simulink subsystem "DriverHEVPowerSplit_refsub"  (R2020b)
settings: Solver=VariableStepAuto  StartTime=0.0  StopTime=10.0  RelTol=1e-3
undefined symbols (not defined in the file or in its folder): driver, initial
libraries: EVComponents_utility_lib x3, simulink x2
settings Model: Creator=isaacito  LastModifiedBy=isaacito

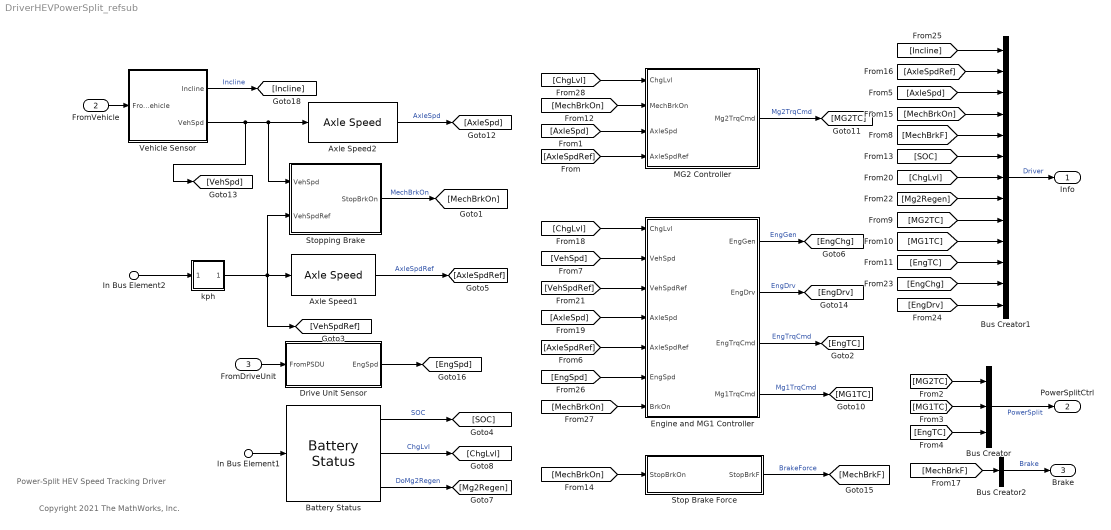
== system DriverHEVPowerSplit_refsub ==
  note: Power-Split HEV Speed Tracking Driver
  note: Copyright 2021 The MathWorks, Inc.
  In Bus Element1 : Inport  PortName=FromBattery  Element=Current
  FromVehicle : Inport  Port=2
  FromDriveUnit : Inport  Port=3
  In Bus Element2 : Inport  Port=4  PortName=FromDrvPattern  Element=VehSpdRef
      settings: AttributesFormatString=%<Unit>
  Axle Speed1 : EVComponents_utility_lib/Axle Speed  Value=driver.tireRadius_m
  Axle Speed2 : EVComponents_utility_lib/Axle Speed  Value=driver.tireRadius_m
  Battery Status : EVComponents_utility_lib/Battery Status  capacity_Ahr=driver.hvbattCapacity_Ahr  initial_SOC_pct=initial.driverHVBattSOC_pct  SocHigh=driver.hvbattSocHighMid_pct  SocLow=driver.hvbattSocMidLow_pct  SocEmpty=driver.hvbattSocLowEmpty_pct
  Bus Creator : BusCreator  Inputs=3
  Bus Creator1 : BusCreator  Inputs=13
  Bus Creator2 : BusCreator  Inputs=1
  Drive Unit Sensor : Subsystem
  Engine and MG1 Controller : Subsystem
  MG2 Controller : Subsystem
  Stop Brake Force : Subsystem
  Stopping Brake : Subsystem
  Vehicle Sensor : Subsystem
  kph : Subsystem
  Info : Outport
  PowerSplitCtrl : Outport  Port=2
  Brake : Outport  Port=3
  wires:
  In Bus Element2/1 -> kph/1(In1)
  FromVehicle/1 -> Vehicle Sensor/1(FromVehicle)
  Vehicle Sensor/2(VehSpd) -> Axle Speed2/1, Stopping Brake/1(VehSpd), [VehSpd]
  Battery Status/1 -> [SOC]  "SOC"
  [SOC] -> Bus Creator1/6
  [Mg2Regen] -> Bus Creator1/8
  [ChgLvl] -> Bus Creator1/7
  [MechBrkOn] -> Bus Creator1/4
  [AxleSpd] -> Bus Creator1/3
  Engine and MG1 Controller/4(Mg1TrqCmd) -> [MG1TC]  "Mg1TrqCmd"
  [VehSpdRef] -> Engine and MG1 Controller/3(VehSpdRef)
  [AxleSpdRef] -> Engine and MG1 Controller/5(AxleSpdRef)
  [AxleSpd] -> Engine and MG1 Controller/4(AxleSpd)
  [AxleSpdRef] -> Bus Creator1/2
  Bus Creator1/1 -> Info/1  "Driver"
  [MG1TC] -> Bus Creator1/10
  [MG2TC] -> Bus Creator1/9
  [MechBrkF] -> Bus Creator1/5
  [EngTC] -> Bus Creator1/11
  [VehSpd] -> Engine and MG1 Controller/2(VehSpd)
  Axle Speed2/1 -> [AxleSpd]  "AxleSpd"
  Battery Status/3 -> [Mg2Regen]  "DoMg2Regen"
  Battery Status/2 -> [ChgLvl]  "ChgLvl"
  Engine and MG1 Controller/3(EngTrqCmd) -> [EngTC]  "EngTrqCmd"
  [ChgLvl] -> Engine and MG1 Controller/1(ChgLvl)
  [EngTC] -> Bus Creator/3
  [MG1TC] -> Bus Creator/2
  [MG2TC] -> Bus Creator/1
  Bus Creator/1 -> PowerSplitCtrl/1  "PowerSplit"
  Axle Speed1/1 -> [AxleSpdRef]  "AxleSpdRef"
  [MechBrkF] -> Bus Creator2/1
  Bus Creator2/1 -> Brake/1  "Brake"
  In Bus Element1/1 -> Battery Status/1
  Engine and MG1 Controller/1(EngGen) -> [EngChg]  "EngGen"
  Engine and MG1 Controller/2(EngDrv) -> [EngDrv]  "EngDrv"
  [EngChg] -> Bus Creator1/12
  [EngDrv] -> Bus Creator1/13
  [EngSpd] -> Engine and MG1 Controller/6(EngSpd)
  [MechBrkOn] -> Engine and MG1 Controller/7(BrkOn)
  FromDriveUnit/1 -> Drive Unit Sensor/1(FromPSDU)
  Drive Unit Sensor/1(EngSpd) -> [EngSpd]
  [MechBrkOn] -> MG2 Controller/2(MechBrkOn)
  [AxleSpd] -> MG2 Controller/3(AxleSpd)
  [AxleSpdRef] -> MG2 Controller/4(AxleSpdRef)
  [MechBrkOn] -> Stop Brake Force/1(StopBrkOn)
  Vehicle Sensor/1(Incline) -> [Incline]  "Incline"
  MG2 Controller/1(Mg2TrqCmd) -> [MG2TC]  "Mg2TrqCmd"
  Stopping Brake/1(StopBrkOn) -> [MechBrkOn]  "MechBrkOn"
  Stop Brake Force/1(StopBrkF) -> [MechBrkF]  "BrakeForce"
  [Incline] -> Bus Creator1/1
  [ChgLvl] -> MG2 Controller/1(ChgLvl)
  kph/1(Out1) -> Axle Speed1/1, [VehSpdRef], Stopping Brake/2(VehSpdRef)

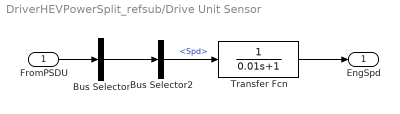
== system DriverHEVPowerSplit_refsub/Drive Unit Sensor ==
  FromPSDU : Inport
  Bus Selector : BusSelector  OutputSignals=eng  OutputAsBus=on
  Bus Selector2 : BusSelector  OutputSignals=Spd
  Transfer Fcn : TransferFcn  Denominator=[0.01 1]
  EngSpd : Outport  Unit=rpm
      settings: AttributesFormatString=%<Unit>
  wires:
  Bus Selector/1 -> Bus Selector2/1
  Transfer Fcn/1 -> EngSpd/1
  FromPSDU/1 -> Bus Selector/1
  Bus Selector2/1 -> Transfer Fcn/1  "<Spd>"

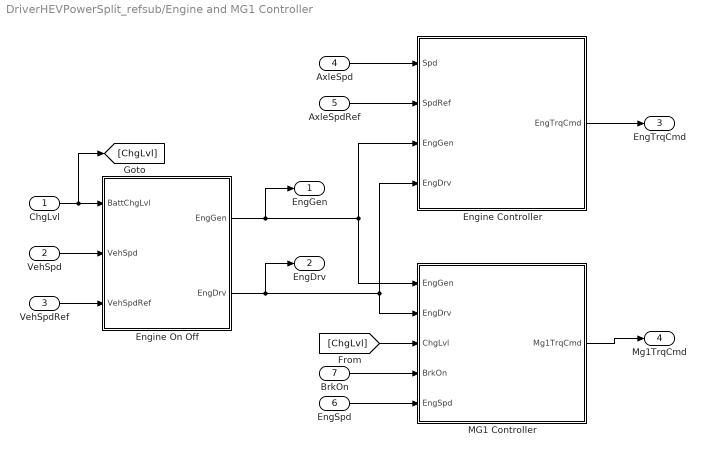
== system DriverHEVPowerSplit_refsub/Engine and MG1 Controller ==
  ChgLvl : Inport
  VehSpd : Inport  Port=2  Unit=km/hr
      settings: AttributesFormatString=%<Unit>
  VehSpdRef : Inport  Port=3  Unit=km/hr
      settings: AttributesFormatString=%<Unit>
  AxleSpd : Inport  Port=4  Unit=rpm
      settings: AttributesFormatString=%<Unit>
  AxleSpdRef : Inport  Port=5  Unit=rpm
      settings: AttributesFormatString=%<Unit>
  EngSpd : Inport  Port=6  Unit=rpm
      settings: AttributesFormatString=%<Unit>
  BrkOn : Inport  Port=7
  Engine Controller : Subsystem
  Engine On Off : Stateflow chart  TreatAsAtomicUnit=on
  MG1 Controller : Subsystem
  EngGen : Outport
  EngDrv : Outport  Port=2
  EngTrqCmd : Outport  Port=3  Unit=N*m
      settings: AttributesFormatString=%<Unit>
  Mg1TrqCmd : Outport  Port=4  Unit=N*m
      settings: AttributesFormatString=%<Unit>
  wires:
  VehSpd/1 -> Engine On Off/2(VehSpd)
  ChgLvl/1 -> [ChgLvl], Engine On Off/1(BattChgLvl)
  VehSpdRef/1 -> Engine On Off/3(VehSpdRef)
  Engine On Off/1(EngGen) -> MG1 Controller/1(EngGen), Engine Controller/3(EngGen), EngGen/1
  Engine On Off/2(EngDrv) -> EngDrv/1, Engine Controller/4(EngDrv), MG1 Controller/2(EngDrv)
  AxleSpd/1 -> Engine Controller/1(Spd)
  AxleSpdRef/1 -> Engine Controller/2(SpdRef)
  Engine Controller/1(EngTrqCmd) -> EngTrqCmd/1
  BrkOn/1 -> MG1 Controller/4(BrkOn)
  EngSpd/1 -> MG1 Controller/5(EngSpd)
  MG1 Controller/1(Mg1TrqCmd) -> Mg1TrqCmd/1
  [ChgLvl] -> MG1 Controller/3(ChgLvl)

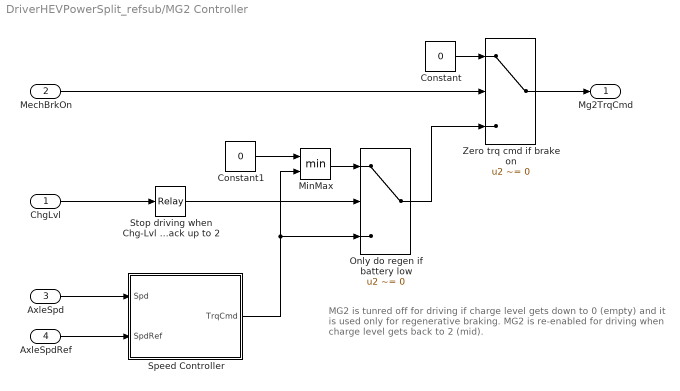
== system DriverHEVPowerSplit_refsub/MG2 Controller ==
  note: MG2 is tunred off for driving if charge level gets down to 0 (empty)
      | and it is used only for regenerative braking.
      | MG2 is re-enabled for driving when charge level gets back to 2 (mid).
  ChgLvl : Inport
  MechBrkOn : Inport  Port=2  OutDataTypeStr=boolean
      settings: AttributesFormatString=%<OutDataTypeStr>
  AxleSpd : Inport  Port=3  Unit=rpm
      settings: AttributesFormatString=%<Unit>
  AxleSpdRef : Inport  Port=4  Unit=rpm
      settings: AttributesFormatString=%<Unit>
  Constant : Constant  Value=0
  Constant1 : Constant  Value=0
  MinMax : MinMax  Inputs=2
  Only do regen if battery low : Switch  Criteria=u2 ~= 0
  Speed Controller : Subsystem
      settings: PortSchema="{\"entries\":[{\"content\":{\"sides\":[{\"content\":{\"connectorIds\":[\"Out1\"]},\"type\":\"ConnectorPlacement.EquallySpacedRectSide\",\"uuid\":\"12b9f2c9-2b28-451b-ad36-7fe4150db485\"},{\"content\":{\"connectorIds\":[\"In1\",\"In2\"],\"side\":\"RIGHT\"},\"type\":\"ConnectorPlacement.EquallySpacedRectSide\",\"uuid\":\"c0fdf9a4-483a-4ddc-b663-6299fcc79327\"},{\"content\":{\"connectorIds\":[],\"side\":\"TOP\"},\"type\":\"ConnectorPlacement.EquallySpacedRectSide\",\"uuid\":\"3f20082e-8487-45e3-9fd7-d6d75741df4d\"}]},\"type\":\"ConnectorPlacement.EquallySpacedConnector\",\"uuid\":\"9361cdd3-74d8-46ee-ae7f-e2dde5d31ed1\"}],\"packageUris\":[\"http://schema.mathworks.com/mf0/Connector/R2020b\"],\"version\":\"1.0\"}"
  Stop driving when Chg-Lvl down to 0 Resume when ChgLvl back up to 2 : Relay  OnSwitchValue=2  OffSwitchValue=0  OnOutputValue=0  OffOutputValue=1
  Zero trq cmd if brake on : Switch  Criteria=u2 ~= 0
  Mg2TrqCmd : Outport  Unit=N*m
      settings: AttributesFormatString=%<Unit>
  wires:
  Constant1/1 -> MinMax/1
  MinMax/1 -> Only do regen if battery low/1
  Only do regen if battery low/1 -> Zero trq cmd if brake on/3
  ChgLvl/1 -> Stop driving when Chg-Lvl down to 0 Resume when ChgLvl back up to 2/1
  Zero trq cmd if brake on/1 -> Mg2TrqCmd/1
  AxleSpdRef/1 -> Speed Controller/2(SpdRef)
  MechBrkOn/1 -> Zero trq cmd if brake on/2
  Constant/1 -> Zero trq cmd if brake on/1
  AxleSpd/1 -> Speed Controller/1(Spd)
  Speed Controller/1(TrqCmd) -> MinMax/2, Only do regen if battery low/3
  Stop driving when Chg-Lvl down to 0 Resume when ChgLvl back up to 2/1 -> Only do regen if battery low/2

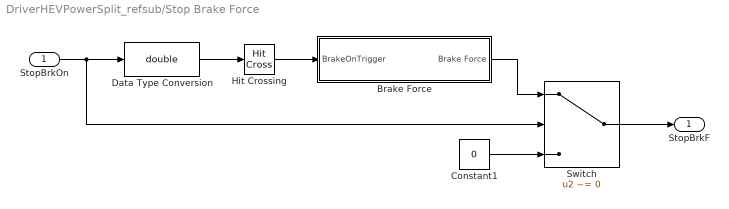
== system DriverHEVPowerSplit_refsub/Stop Brake Force ==
  StopBrkOn : Inport  OutDataTypeStr=boolean
      settings: AttributesFormatString=%<OutDataTypeStr>
  Brake Force : Subsystem  TreatAsAtomicUnit=on
  Constant1 : Constant  Value=0
  Data Type Conversion : DataTypeConversion  OutDataTypeStr=double
  Hit Crossing : HitCross  HitCrossingOffset=0.5  HitCrossingDirection=rising
      settings: AttributesFormatString=%<HitCrossingOffset>
  Switch : Switch  Criteria=u2 ~= 0  Threshold=0.5
  StopBrkF : Outport  Unit=N
      settings: AttributesFormatString=%<Unit>
  wires:
  Data Type Conversion/1 -> Hit Crossing/1
  StopBrkOn/1 -> Data Type Conversion/1, Switch/2
  Hit Crossing/1 -> Brake Force/1(BrakeOnTrigger)
  Brake Force/1(Brake Force) -> Switch/1
  Switch/1 -> StopBrkF/1
  Constant1/1 -> Switch/3

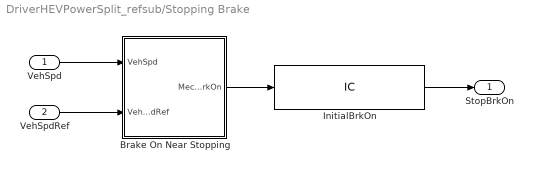
== system DriverHEVPowerSplit_refsub/Stopping Brake ==
  VehSpd : Inport
      settings: AttributesFormatString=%<Unit>
  VehSpdRef : Inport  Port=2
      settings: AttributesFormatString=%<Unit>
  Brake On Near Stopping : Stateflow chart  TreatAsAtomicUnit=on
  InitialBrkOn : InitialCondition  Value=initial.driverBrakeOn_tf
  StopBrkOn : Outport  OutDataTypeStr=boolean
      settings: AttributesFormatString=%<OutDataTypeStr>
  wires:
  InitialBrkOn/1 -> StopBrkOn/1
  VehSpdRef/1 -> Brake On Near Stopping/2(VehSpdRef)
  Brake On Near Stopping/1(MechBrkOn) -> InitialBrkOn/1
  VehSpd/1 -> Brake On Near Stopping/1(VehSpd)

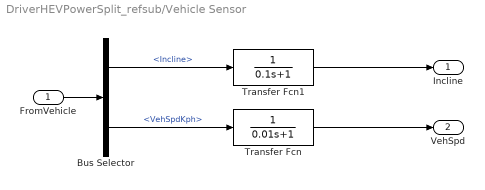
== system DriverHEVPowerSplit_refsub/Vehicle Sensor ==
  FromVehicle : Inport
  Bus Selector : BusSelector  OutputSignals=Incline,VehSpdKph
  Transfer Fcn : TransferFcn  Denominator=[0.01 1]
  Transfer Fcn1 : TransferFcn  Denominator=[0.1 1]
  Incline : Outport  Unit=deg
      settings: AttributesFormatString=%<Unit>
  VehSpd : Outport  Port=2  Unit=km/hr
      settings: AttributesFormatString=%<Unit>
  wires:
  Transfer Fcn1/1 -> Incline/1
  Bus Selector/1 -> Transfer Fcn1/1  "<Incline>"
  Transfer Fcn/1 -> VehSpd/1
  FromVehicle/1 -> Bus Selector/1
  Bus Selector/2 -> Transfer Fcn/1  "<VehSpdKph>"

== system DriverHEVPowerSplit_refsub/kph ==
  In1 : Inport
  Signal Specification : SignalSpecification  Unit=km/hr
  Unit Conversion : UnitConversion
  Out1 : Outport
  wires:
  Signal Specification/1 -> Out1/1
  In1/1 -> Unit Conversion/1
  Unit Conversion/1 -> Signal Specification/1

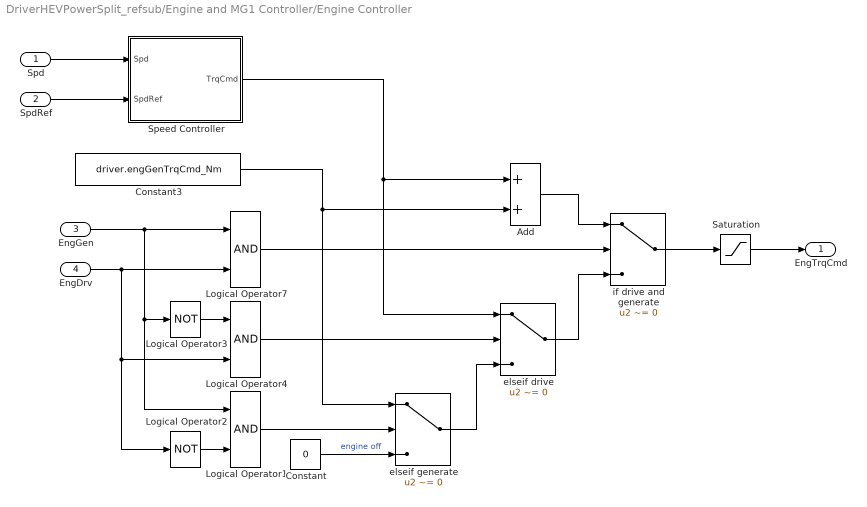
== system DriverHEVPowerSplit_refsub/Engine and MG1 Controller/Engine Controller ==
  Spd : Inport  Unit=rpm
      settings: AttributesFormatString=%<Unit>
  SpdRef : Inport  Port=2  Unit=rpm
      settings: AttributesFormatString=%<Unit>
  EngGen : Inport  Port=3
  EngDrv : Inport  Port=4
  Add : Sum
  Constant : Constant  Value=0
  Constant3 : Constant  Value=driver.engGenTrqCmd_Nm
  Logical Operator1 : Logic  AllPortsSameDT=off  OutDataTypeStr=boolean
  Logical Operator2 : Logic  Operator=NOT  AllPortsSameDT=off  OutDataTypeStr=boolean
  Logical Operator3 : Logic  Operator=NOT  AllPortsSameDT=off  OutDataTypeStr=boolean
  Logical Operator4 : Logic  AllPortsSameDT=off  OutDataTypeStr=boolean
  Logical Operator7 : Logic  AllPortsSameDT=off  OutDataTypeStr=boolean
  Saturation : Saturate  UpperLimit=driver.engTrqMax_Nm  LowerLimit=0
      settings: AttributesFormatString=|
      | %<UpperLimit>
      | %<LowerLimit>
  Speed Controller : Subsystem
      settings: PortSchema="{\"entries\":[{\"content\":{\"sides\":[{\"content\":{\"connectorIds\":[\"Out1\"]},\"type\":\"ConnectorPlacement.EquallySpacedRectSide\",\"uuid\":\"12b9f2c9-2b28-451b-ad36-7fe4150db485\"},{\"content\":{\"connectorIds\":[\"In1\",\"In2\"],\"side\":\"RIGHT\"},\"type\":\"ConnectorPlacement.EquallySpacedRectSide\",\"uuid\":\"c0fdf9a4-483a-4ddc-b663-6299fcc79327\"},{\"content\":{\"connectorIds\":[],\"side\":\"TOP\"},\"type\":\"ConnectorPlacement.EquallySpacedRectSide\",\"uuid\":\"3f20082e-8487-45e3-9fd7-d6d75741df4d\"}]},\"type\":\"ConnectorPlacement.EquallySpacedConnector\",\"uuid\":\"9361cdd3-74d8-46ee-ae7f-e2dde5d31ed1\"}],\"packageUris\":[\"http://schema.mathworks.com/mf0/Connector/R2020b\"],\"version\":\"1.0\"}"
  elseif drive : Switch  Criteria=u2 ~= 0
  elseif generate : Switch  Criteria=u2 ~= 0
  if drive and generate : Switch  Criteria=u2 ~= 0
  EngTrqCmd : Outport  Unit=N*m
      settings: AttributesFormatString=%<Unit>
  wires:
  if drive and generate/1 -> Saturation/1
  Constant/1 -> elseif generate/3  "engine off"
  elseif generate/1 -> elseif drive/3
  Logical Operator1/1 -> elseif generate/2
  Logical Operator4/1 -> elseif drive/2
  elseif drive/1 -> if drive and generate/3
  Add/1 -> if drive and generate/1
  Logical Operator7/1 -> if drive and generate/2
  Logical Operator3/1 -> Logical Operator4/1
  EngGen/1 -> Logical Operator1/1, Logical Operator3/1, Logical Operator7/1
  Logical Operator2/1 -> Logical Operator1/2
  EngDrv/1 -> Logical Operator7/2, Logical Operator2/1, Logical Operator4/2
  Saturation/1 -> EngTrqCmd/1
  Spd/1 -> Speed Controller/1(Spd)
  SpdRef/1 -> Speed Controller/2(SpdRef)
  Speed Controller/1(TrqCmd) -> Add/1, elseif drive/1
  Constant3/1 -> Add/2, elseif generate/1

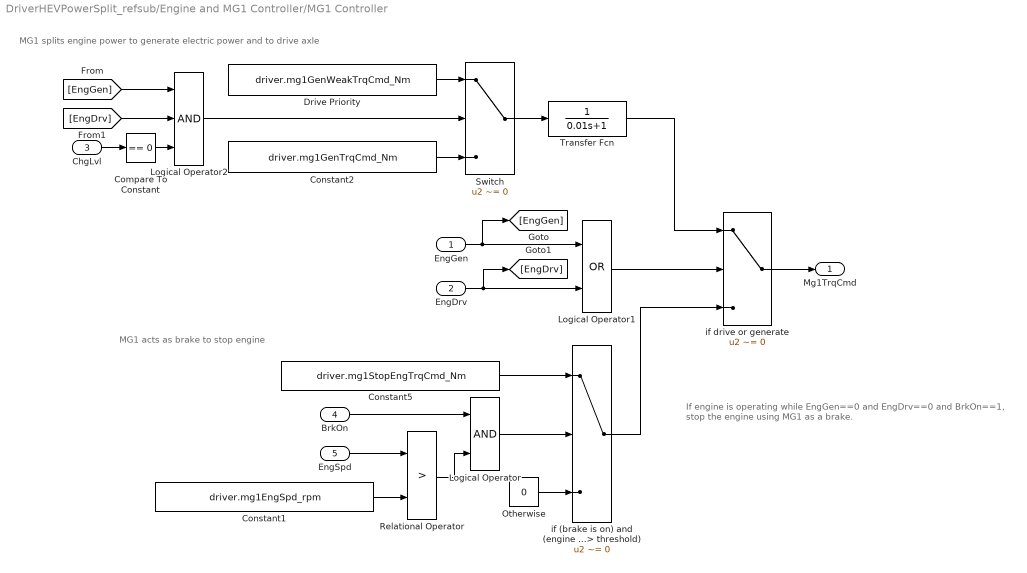
== system DriverHEVPowerSplit_refsub/Engine and MG1 Controller/MG1 Controller ==
  note: If engine is operating
      | while EngGen==0 and EngDrv==0 and BrkOn==1,
      | stop the engine using MG1 as a brake.
  note: MG1 acts as brake to stop engine
  note: MG1 splits engine power to generate electric power and to drive axle
  EngGen : Inport
  EngDrv : Inport  Port=2
  ChgLvl : Inport  Port=3
  BrkOn : Inport  Port=4
  EngSpd : Inport  Port=5  Unit=rpm
      settings: AttributesFormatString=%<Unit>
  Compare To Constant : simulink/Logic and Bit Operations/Compare To Constant  relop===  const=0  OutDataTypeStr=boolean
  Constant1 : Constant  Value=driver.mg1EngSpd_rpm
  Constant2 : Constant  Value=driver.mg1GenTrqCmd_Nm
  Constant5 : Constant  Value=driver.mg1StopEngTrqCmd_Nm
  Drive Priority : Constant  Value=driver.mg1GenWeakTrqCmd_Nm
  Logical Operator : Logic  AllPortsSameDT=off  OutDataTypeStr=boolean
  Logical Operator1 : Logic  Operator=OR  AllPortsSameDT=off  OutDataTypeStr=boolean
  Logical Operator2 : Logic  Inputs=3  AllPortsSameDT=off  OutDataTypeStr=boolean
  Otherwise : Constant  Value=0
  Relational Operator : RelationalOperator  Operator=>  OutDataTypeStr=boolean  RndMeth=Simplest
  Switch : Switch  Criteria=u2 ~= 0
  Transfer Fcn : TransferFcn  Denominator=[0.01 1]
  if (brake is on) and (engine speed > threshold) : Switch  Criteria=u2 ~= 0
  if drive or generate : Switch  Criteria=u2 ~= 0
  Mg1TrqCmd : Outport  Unit=N*m
      settings: AttributesFormatString=%<Unit>
  wires:
  Compare To Constant/1 -> Logical Operator2/3
  Logical Operator1/1 -> if drive or generate/2
  Transfer Fcn/1 -> if drive or generate/1
  Switch/1 -> Transfer Fcn/1
  Constant1/1 -> Relational Operator/2
  BrkOn/1 -> Logical Operator/1
  Constant5/1 -> if (brake is on) and (engine speed > threshold)/1
  Relational Operator/1 -> Logical Operator/2
  Logical Operator/1 -> if (brake is on) and (engine speed > threshold)/2
  if (brake is on) and (engine speed > threshold)/1 -> if drive or generate/3
  EngGen/1 -> [EngGen], Logical Operator1/1
  EngSpd/1 -> Relational Operator/1
  Otherwise/1 -> if (brake is on) and (engine speed > threshold)/3
  EngDrv/1 -> [EngDrv], Logical Operator1/2
  if drive or generate/1 -> Mg1TrqCmd/1
  [EngGen] -> Logical Operator2/1
  [EngDrv] -> Logical Operator2/2
  Logical Operator2/1 -> Switch/2
  Constant2/1 -> Switch/3
  Drive Priority/1 -> Switch/1
  ChgLvl/1 -> Compare To Constant/1

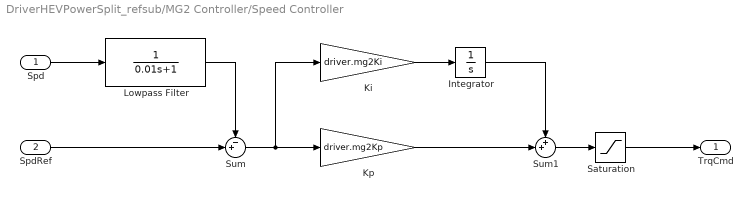
== system DriverHEVPowerSplit_refsub/MG2 Controller/Speed Controller ==
  Spd : Inport  Unit=rpm
      settings: AttributesFormatString=%<Unit>
  SpdRef : Inport  Port=2  Unit=rpm
      settings: AttributesFormatString=%<Unit>
  Integrator : Integrator  LimitOutput=on  UpperSaturationLimit=driver.mg2TrqMax_Nm  LowerSaturationLimit=-driver.mg2TrqMax_Nm
      settings: AttributesFormatString=|
      | %<UpperSaturationLimit>
      | %<LowerSaturationLimit>
  Ki : Gain  Gain=driver.mg2Ki
  Kp : Gain  Gain=driver.mg2Kp
  Lowpass Filter : TransferFcn  Denominator=[0.01 1]
  Saturation : Saturate  UpperLimit=driver.mg2TrqMax_Nm  LowerLimit=-driver.mg2TrqMax_Nm
      settings: AttributesFormatString=|
      | %<UpperLimit>
      | %<LowerLimit>
  Sum : Sum  Inputs=-+|
  Sum1 : Sum  Inputs=++|
  TrqCmd : Outport  Unit=N*m  VectorParamsAs1DForOutWhenUnconnected=off
      settings: AttributesFormatString=%<Unit>
  wires:
  Lowpass Filter/1 -> Sum/1
  Spd/1 -> Lowpass Filter/1
  Integrator/1 -> Sum1/1
  Kp/1 -> Sum1/2
  Ki/1 -> Integrator/1
  Sum/1 -> Ki/1, Kp/1
  Sum1/1 -> Saturation/1
  SpdRef/1 -> Sum/2
  Saturation/1 -> TrqCmd/1

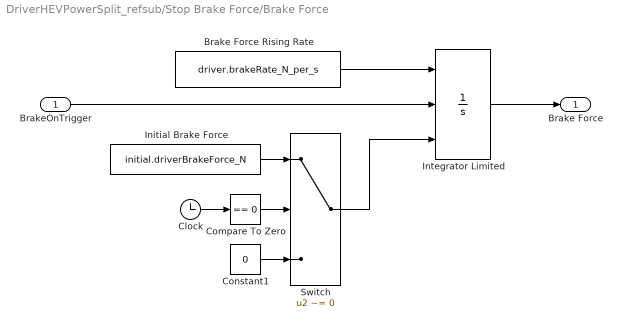
== system DriverHEVPowerSplit_refsub/Stop Brake Force/Brake Force ==
  BrakeOnTrigger : Inport
  Brake Force Rising Rate : Constant  Value=driver.brakeRate_N_per_s
  Clock : Clock
  Compare To Zero : simulink/Logic and Bit Operations/Compare To Zero  relop===  OutDataTypeStr=boolean
  Constant1 : Constant  Value=0
  Initial Brake Force : Constant  Value=initial.driverBrakeForce_N
  Integrator Limited : Integrator  ExternalReset=rising  InitialConditionSource=external  LimitOutput=on  UpperSaturationLimit=driver.brakeForceMax_N  LowerSaturationLimit=0
      settings: AttributesFormatString=%<UpperSaturationLimit>
  Switch : Switch  Criteria=u2 ~= 0
  Brake Force : Outport  Unit=N
      settings: AttributesFormatString=%<Unit>
  wires:
  Brake Force Rising Rate/1 -> Integrator Limited/1
  Constant1/1 -> Switch/3
  Switch/1 -> Integrator Limited/3
  Initial Brake Force/1 -> Switch/1
  Compare To Zero/1 -> Switch/2
  Clock/1 -> Compare To Zero/1
  Integrator Limited/1 -> Brake Force/1
  BrakeOnTrigger/1 -> Integrator Limited/2

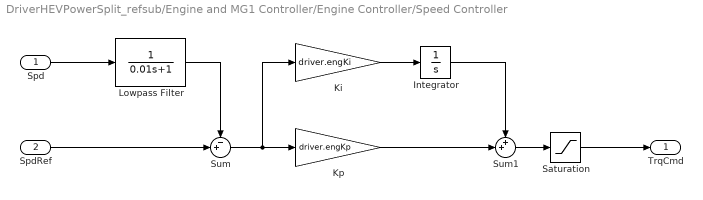
== system DriverHEVPowerSplit_refsub/Engine and MG1 Controller/Engine Controller/Speed Controller ==
  Spd : Inport  Unit=rpm
      settings: AttributesFormatString=%<Unit>
  SpdRef : Inport  Port=2  Unit=rpm
      settings: AttributesFormatString=%<Unit>
  Integrator : Integrator  LimitOutput=on  UpperSaturationLimit=driver.engTrqMax_Nm  LowerSaturationLimit=0
      settings: AttributesFormatString=%<UpperSaturationLimit>
  Ki : Gain  Gain=driver.engKi
  Kp : Gain  Gain=driver.engKp
  Lowpass Filter : TransferFcn  Denominator=[0.01 1]
  Saturation : Saturate  UpperLimit=driver.engTrqMax_Nm  LowerLimit=0
      settings: AttributesFormatString=|
      | %<UpperLimit>
      | %<LowerLimit>
  Sum : Sum  Inputs=-+|
  Sum1 : Sum  Inputs=++|
  TrqCmd : Outport  Unit=N*m  VectorParamsAs1DForOutWhenUnconnected=off
      settings: AttributesFormatString=%<Unit>
  wires:
  SpdRef/1 -> Sum/2
  Spd/1 -> Lowpass Filter/1
  Sum1/1 -> Saturation/1
  Sum/1 -> Ki/1, Kp/1
  Ki/1 -> Integrator/1
  Kp/1 -> Sum1/2
  Integrator/1 -> Sum1/1
  Lowpass Filter/1 -> Sum/1
  Saturation/1 -> TrqCmd/1

== stateflow chart DriverHEVPowerSplit_refsub/Stopping Brake/Brake On Near Stopping ==
  state Initial
  state BrakeOn
    entry:
    MechBrkOn = true;
  state BrakeOff
    entry:
    MechBrkOn = false;
  (default) -> Initial
  Initial -> (junction 22) [order 2] : [abs(VehSpd) <= BrkOnSpd]
  Initial -> (junction 24) [order 1] : [ BrkOnSpd < VehSpd ...
      |  || VehSpd < -BrkOnSpd]
  (junction 22) -> BrakeOn
  (junction 24) -> BrakeOff
  BrakeOn -> BrakeOff : [ VehSpdRef > 0.01 ...
      |  && (BrkOffDeltaSpd < VehSpdRef - VehSpd...
      |       || VehSpdRef - VehSpd < -BrkOffDeltaSpd ) ]
  BrakeOff -> BrakeOn : [ abs(VehSpd) < BrkOnSpd ...
      |  && abs(VehSpdRef) < 0.001 ]
  data: VehSpd input; MechBrkOn output; VehSpdRef input; BrkOnSpd local =driver.brakeOnSpd_kph; BrkOffDeltaSpd local =driver.brakeOffSpdDiff_kph

== stateflow chart DriverHEVPowerSplit_refsub/Engine and MG1 Controller/Engine On Off ==
  state Initial
  state EngineOff
    entry:
    EngDrv = false;
    EngGen = false;
  state EngineDriveGenerate
    entry:
    EngDrv = true;
    EngGen = true;
  state EngineDrive
    entry:
    EngDrv = true;
    EngGen = false;
  state EngineGenerate
    entry:
    EngDrv = false;
    EngGen = true;
  (default) -> Initial
  Initial -> (junction 34) [order 2] : [ (BattChgLvl == 2 || BattChgLvl == 3) ...
      |  && VehSpdRef < engOnVehSpd ]
  Initial -> (junction 36) [order 1] : [ BattChgLvl == 1 ...
      |  && 0.01 < VehSpdRef ]
  (junction 34) -> EngineOff
  (junction 36) -> EngineDriveGenerate
  Initial -> (junction 42) [order 4] : [ (BattChgLvl == 2 || BattChgLvl == 3) ...
      |  && engOnVehSpd <= VehSpdRef ]
  (junction 42) -> EngineDrive
  Initial -> EngineGenerate [order 3] : [ BattChgLvl == 0 ...
      |   || (BattChgLvl == 1 ...
      |        && VehSpdRef < 0.01) ]
  (junction 30) -> EngineOff
  EngineDriveGenerate -> (junction 30) [order 3] : [ BattChgLvl == 3 ...
      |  && VehSpd < engOnVehSpd - 10 ]
  (junction 50) -> EngineOff : [ (BattChgLvl == 2 || BattChgLvl == 3) ...
      |   && VehSpd < engOnVehSpd - 10 ]
  EngineDrive -> (junction 50) [order 1]
  EngineOff -> (junction 54) [order 1]
  (junction 46) -> EngineOff
  EngineOff -> (junction 44) [order 2] : [ (BattChgLvl == 0 ...
      |     || BattChgLvl == 1) ...
      |  || (BattChgLvl == 2 ...
      |      && chgSpd < VehSpd) ]
  (junction 54) -> EngineDrive : [ (BattChgLvl == 2 || BattChgLvl == 3) ...
      |   && engOnVehSpd < VehSpd ...
      |   && VehSpd < VehSpdRef + 0.1 ]
  EngineDriveGenerate -> EngineDrive [order 2] : [ BattChgLvl == 3 ...
      | && engOnVehSpd - 10 < VehSpd ]
  EngineDrive -> EngineDriveGenerate [order 2] : [ BattChgLvl == 1 ...
      | || (BattChgLvl == 2 ...
      |      && chgSpd < VehSpd) ]
  (junction 38) -> EngineDriveGenerate
  EngineDriveGenerate -> (junction 40) [order 1] : [ BattChgLvl == 0 ...
      | || ((BattChgLvl == 1 || BattChgLvl == 2) ...
      |      && abs(VehSpd) < 0.01) ]
  (junction 48) -> EngineDrive
  (junction 40) -> EngineGenerate
  EngineGenerate -> (junction 48) [order 1] : [ BattChgLvl == 3 ...
      |  && engOnVehSpd < VehSpd ]
  EngineGenerate -> (junction 46) [order 2] : [ BattChgLvl == 3 ...
      |  && VehSpd < engOnVehSpd ]
  EngineGenerate -> (junction 38) [order 3] : [ (BattChgLvl == 1 || BattChgLvl == 2) ...
      |  && 1 < VehSpdRef ]
  (junction 44) -> EngineGenerate
  data: BattChgLvl input; VehSpd input; engOnVehSpd constant double =driver.engOnVehSpd_kph; EngGen output; EngDrv output; VehSpdRef input; chgSpd constant double =driver.chgSpd_kph
